simulink model "Radial_LV_Grid_CVR"  (R2022a)
settings: Solver=ode23t  StartTime=0.0  StopTime=10  MaxStep=0.1  RelTol=1e-3
libraries: spsLoadFlowBusLib x3, spsThreePhaseVIMeasurementLib x3, spsPower3phPhasorLib x2, spsThreePhasePISectionLineLib x1, spsThreePhaseDynamicLoadLib x1, spsThreePhaseProgrammableVoltageSourceLib x1, spsThreePhaseTransformerTwoWindingsLib x1, spspowerguiLib x1
settings Model: Creator=matm  LastModifiedBy=nikos
settings SolverCC: ShapePreserveControl=EnableAll  AlgebraicLoopSolver=TrustRegion  SolverResetMethod=Robust
settings DataIOCC: ReturnWorkspaceOutputs=off
settings DebuggingCC: SFMachineParentedDataDiag=warning  ArithmeticOperatorsInVariantConditions=warning
settings SFSimCC: SimUseLocalCustomCode=off  CustomCodeUndefinedFunction=UseInterfaceOnly
settings RTWCC: RTWUseLocalCustomCode=off
settings CodeAppCC: StateflowObjectComments=on
settings SimscapeCC: SimscapeNormalizeSystem=off

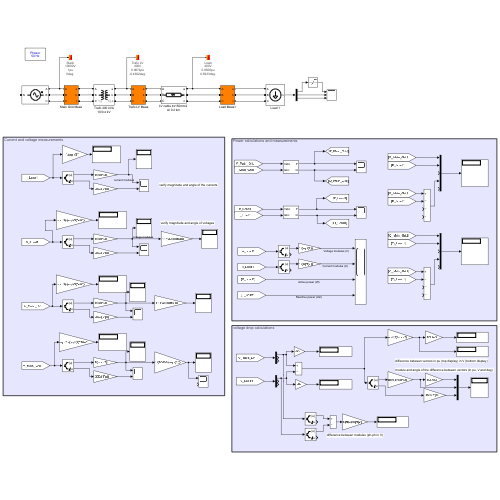
[thumbnail: Simulink's stored preview of the top-level diagram]
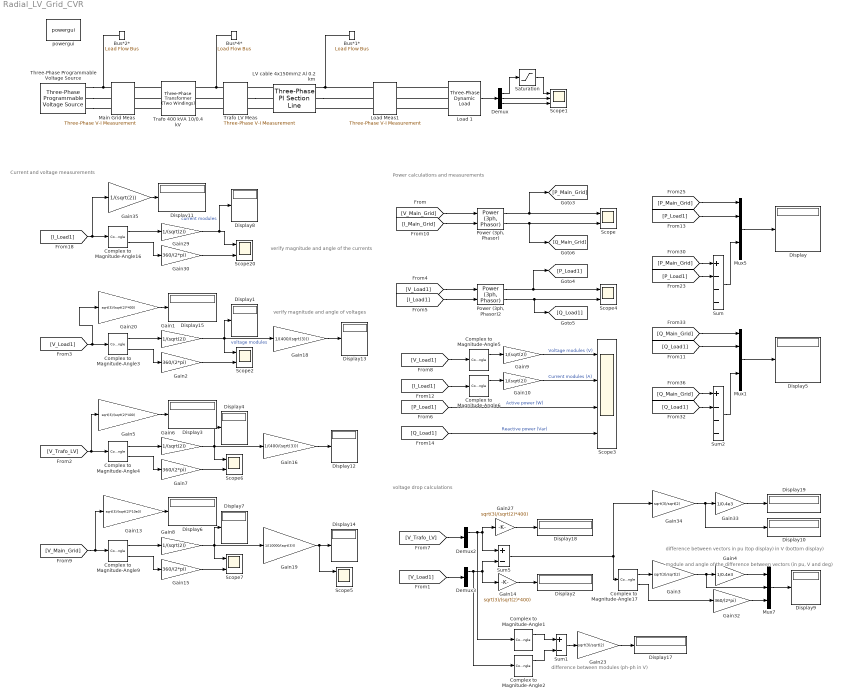
== system Radial_LV_Grid_CVR ==
  note: Power calculations and measurements
  note: voltage drop calculations
  note: difference between vectors in pu (top display) in V (bottom display)
  note: verify magnitude and angle of voltages
  note: verify magnitude and angle of the currents
  note: Current and voltage measurements
  note: difference between modules (ph-ph in V)
  note: module and angle of the difference between vectors (in pu, V and deg)
  Bus*1* : spsLoadFlowBusLib/Load Flow Bus  LConnTagsString=a  Phases=single  Connectors=on one side  ID=Load  Vbase=400  Vref=1  Vangle=0  VLF=0.9506  VLFb=1  VLFc=1  angleLF=0.5933  angleLFb=0  angleLFc=0
      settings: SourceProductBaseCode=PS
  Bus*2* : spsLoadFlowBusLib/Load Flow Bus  LConnTagsString=a  Phases=single  Connectors=on one side  ID=Slack  Vbase=10000  Vref=1  Vangle=0  VLF=1  VLFb=1  VLFc=1  angleLF=0  angleLFb=0  angleLFc=0
      settings: SourceProductBaseCode=PS
  Bus*4* : spsLoadFlowBusLib/Load Flow Bus  LConnTagsString=a  Phases=single  Connectors=on one side  ID=Trafo LV  Vbase=400  Vref=1  Vangle=0  VLF=0.9874  VLFb=1  VLFc=1  angleLF=-0.4362  angleLFb=0  angleLFc=0
      settings: SourceProductBaseCode=PS
  Complex to Magnitude-Angle{1..6,9,16..17} (9 alike) : ComplexToMagnitudeAngle
  Demux : Demux  Outputs=3
  Demux2 : Demux  Outputs=3
  Demux3 : Demux  Outputs=3
  Display{,1..15,17..19} (19 alike) : Display
  Gain{1,6,8..10,29,35} (7 alike) : Gain  Gain=1/(sqrt(2))
  Gain13 : Gain  Gain=sqrt(3)/(sqrt(2)*10e3)
  Gain{5,14,20,27} (4 alike) : Gain  Gain=sqrt(3)/(sqrt(2)*400)
  Gain{2,7,15,30,32} (5 alike) : Gain  Gain=360/(2*pi)
  Gain16 : Gain  Gain=1/(400/(sqrt(3)))
  Gain18 : Gain  Gain=1/(400/(sqrt(3)))
  Gain19 : Gain  Gain=1/(10000/(sqrt(3)))
  Gain23 : Gain  Gain=sqrt(3)/sqrt(2)
  Gain3 : Gain  Gain=sqrt(3)/sqrt(2)
  Gain33 : Gain  Gain=1/0.4e3
  Gain34 : Gain  Gain=sqrt(3)/sqrt(2)
  Gain4 : Gain  Gain=1/0.4e3
  LV cable 4x150mm2 Al 0.2 km : spsThreePhasePISectionLineLib/Three-Phase PI Section Line  LConnTagsString=a|b|c  RConnTagsString=A|B|C  Length=0.2  Frequency=50  Resistances=[ 0.207 0.83]  Inductances=[ 72e-3/(2*pi*50) 289e-3/(2*pi*50)]  Capacitances=[910e-09 411e-09]
  Load 1 : spsThreePhaseDynamicLoadLib/Three-Phase Dynamic Load  NominalVoltage=[ 0.4e3 50 ]  ActiveReactivePowers=[100000 100000]  PositiveSequence=[0.950611 0.593329]  ExternalControl=off  NpNq=[2 2]  TimeConstants="[0  0  0  0]"  MinimumVoltage=0.7  Tfilter=1e-4  LoadFlowParameters=[4 100000 0 0 100000]
      settings: SourceProductBaseCode=PS
  Load Meas1 : spsThreePhaseVIMeasurementLib/Three-Phase V-I Measurement  VoltageMeasurement=phase-to-ground  SetLabelV=on  LabelV=V_Load1  Vpu=off  VpuLL=off  CurrentMeasurement=yes  SetLabelI=on  LabelI=I_Load1  Ipu=off  Pbase=100e6  Vbase=500e3  OutputType=Complex  PhasorSimulation=on  PSBequivalent=0
  Main Grid Meas : spsThreePhaseVIMeasurementLib/Three-Phase V-I Measurement  VoltageMeasurement=phase-to-ground  SetLabelV=on  LabelV=V_Main_Grid  Vpu=off  VpuLL=off  CurrentMeasurement=yes  SetLabelI=on  LabelI=I_Main_Grid  Ipu=off  Pbase=100e6  Vbase=500e3  OutputType=Complex  PhasorSimulation=on  PSBequivalent=0
  Mux1 : Mux  Inputs=5
  Mux5 : Mux  Inputs=5
  Mux7 : Mux  Inputs=3
  "Power (3ph, Phasor)" : spsPower3phPhasorLib/Power (3ph, Phasor)
      settings: SourceProductBaseCode=PS
  "Power (3ph, Phasor)2" : spsPower3phPhasorLib/Power (3ph, Phasor)
      settings: SourceProductBaseCode=PS
  Saturation : Saturate  UpperLimit=1.15  LowerLimit=0.85
  Scope{,2,4..7,20} (7 alike) : Scope  NumInputPorts=2
  Scope1 : Scope  NumInputPorts=3
  Scope3 : Scope  NumInputPorts=4
  Sum : Sum  Inputs=+---
  Sum1 : Sum  Inputs=+-
  Sum2 : Sum  Inputs=+---
  Sum5 : Sum  Inputs=+-
  Three-Phase Programmable Voltage Source : spsThreePhaseProgrammableVoltageSourceLib/Three-Phase Programmable Voltage Source  PositiveSequence=[(10000)*1 0 50]  VariationEntity=Amplitude  VariationType=Table of time-amplitude pairs  VariationTypeAlt=Step  VariationStep=0.5  VariationRate=10  VariationMagnitude=0.3  VariationFrequency=2  VariationTiming=[1 2]  VariationPhaseA=off  Amplitudes=[1 0.99 0.98 0.97 0.96 0.95]  TimeValues=[0 1 2 3 4 5]  HarmonicGeneration=off  HarmonicA=[3 0.2 -25 0]  HarmonicB=[2 0.15 35 2]  Timing="[0.05  3]"  BusType=swing  Pref=0  Qref=0  Qmin=-inf  Qmax=inf
  Trafo 400 kVA 10/0.4 kV : spsThreePhaseTransformerTwoWindingsLib/Three-Phase Transformer (Two Windings)  Winding1Connection=Yg  Winding2Connection=Yg  CoreType=Three single-phase transformers  SetSaturation=off  Hysteresis=off  DataFile='hysteresis'  SetInitialFlux=off  Measurements=None  UNITS=pu  NominalPower=[ 400e3 , 50 ]  Winding1=[10000 0.005 0.019]  Winding2=[400 0.005 0.019]  Rm=500  Lm=500  L0=0.5  Saturation=[0 0;0.0024 1.2;1 1.52]  InitialFluxes=[0.8 -0.8 0.7]  BreakLoop=off  DiscreteSolver=Trapezoidal iterative  DataType=off  TransfoNumber=1
  Trafo LV Meas : spsThreePhaseVIMeasurementLib/Three-Phase V-I Measurement  VoltageMeasurement=phase-to-ground  SetLabelV=on  LabelV=V_Trafo_LV  Vpu=off  VpuLL=off  CurrentMeasurement=yes  SetLabelI=on  LabelI=I_Trafo_LV  Ipu=off  Pbase=100e6  Vbase=500e3  OutputType=Complex  PhasorSimulation=on  PSBequivalent=0
  powergui : spspowerguiLib/powergui  Priority=1  SimulationMode=Phasor  SampleTime=50e-6  frequency=50  Iterations=50  frequencyindice=50  Pbase=1e6  ErrMax=0.0001  UnitsV=kV  UnitsW=kW  buscounter=7  FunctionMessages=off  echomessages=off  EnableUseOfTLC=off  CurrentSourceSwitches=off  DisableSnubberDevices=off  DisableRonSwitches=off  DisableVfSwitches=off  DisplayEquations=off  AutomaticDiscreteSolvers=off  SolverType=Tustin/Backward Euler (TBE)  Interpol=off  ExternalGateDelay=off  methode=off  Ts=10  x0status=blocks  SPID=off  SwTol=0  HookPort=off  NonlinearTolerance=1e-4  nMaxIteration=100  ContinueOnMaxIteration=off  RestoreLinks=warning  ResistiveCurrentMeasurement=off  Frange=[0:2:500]  Ylog=off  Xlog=on  ShowGrid=off  save=off  variable=ZData  structure=ScopeData  ZoomFFT=off  StartTime=0.0  cycles=1  DisplayStyle=1  fundamental=60  FreqAxis=off  MaxFrequency=1000  frequencyindicesteady=1  RmsSteady=2  display=off
  wires:
  Load 1/1 -> Demux/1
  Demux/3 -> Scope1/3
  Demux/2 -> Scope1/2
  Demux/1 -> Saturation/1
  Saturation/1 -> Scope1/1
  "Power (3ph, Phasor)2"/1 -> [P_Load1], Scope4/1
  Sum2/1 -> Mux1/4
  [P_Main_Grid] -> Sum/1
  [P_Load1] -> Mux5/2
  Mux5/1 -> Display/1
  Gain27/1 -> Display18/1
  [P_Main_Grid] -> Mux5/1
  Sum/1 -> Mux5/4
  [Q_Load1] -> Sum2/2
  [Q_Main_Grid] -> Sum2/1
  [Q_Main_Grid] -> Mux1/1
  [Q_Load1] -> Mux1/2
  Mux1/1 -> Display5/1
  Complex to Magnitude-Angle3/2 -> Gain2/1
  [V_Main_Grid] -> Gain13/1, Complex to Magnitude-Angle9/1
  Gain3/1 -> Mux7/2, Gain4/1
  Complex to Magnitude-Angle9/2 -> Gain15/1
  Gain18/1 -> Display13/1
  Gain20/1 -> Display15/1
  Gain32/1 -> Mux7/3
  [P_Load1] -> Sum/2
  Gain23/1 -> Display17/1
  [V_Trafo_LV] -> Complex to Magnitude-Angle4/1, Gain5/1
  Gain33/1 -> Display19/1
  Sum1/1 -> Gain23/1
  Gain6/1 -> Gain16/1, Scope6/1, Display4/1
  Gain4/1 -> Mux7/1
  Demux2/1 -> Sum5/1, Gain27/1, Complex to Magnitude-Angle1/1
  Gain8/1 -> Scope7/1, Gain19/1, Display7/1
  Gain15/1 -> Scope7/2
  Gain14/1 -> Display2/1
  "Power (3ph, Phasor)"/1 -> Scope/1, [P_Main_Grid]
  Gain5/1 -> Display3/1
  Complex to Magnitude-Angle3/1 -> Gain1/1
  Gain19/1 -> Scope5/1, Display14/1
  Gain13/1 -> Display6/1
  [V_Load1] -> Complex to Magnitude-Angle3/1, Gain20/1
  [I_Load1] -> "Power (3ph, Phasor)2"/2
  Gain29/1 -> Scope20/1, Display8/1  "current modules"
  [V_Load1] -> Demux3/1
  Gain2/1 -> Scope2/2
  [I_Main_Grid] -> "Power (3ph, Phasor)"/2
  Complex to Magnitude-Angle2/1 -> Sum1/2
  Complex to Magnitude-Angle16/1 -> Gain29/1
  Gain7/1 -> Scope6/2
  Gain1/1 -> Scope2/1, Gain18/1, Display1/1  "voltage modules"
  Gain30/1 -> Scope20/2
  Complex to Magnitude-Angle17/2 -> Gain32/1
  Complex to Magnitude-Angle4/2 -> Gain7/1
  Mux7/1 -> Display9/1
  [V_Main_Grid] -> "Power (3ph, Phasor)"/1
  Complex to Magnitude-Angle4/1 -> Gain6/1
  Demux3/1 -> Gain14/1, Sum5/2, Complex to Magnitude-Angle2/1
  Complex to Magnitude-Angle1/1 -> Sum1/1
  Complex to Magnitude-Angle16/2 -> Gain30/1
  Gain35/1 -> Display11/1
  Gain16/1 -> Display12/1
  Gain34/1 -> Gain33/1, Display10/1
  Complex to Magnitude-Angle9/1 -> Gain8/1
  [V_Trafo_LV] -> Demux2/1
  "Power (3ph, Phasor)2"/2 -> [Q_Load1], Scope4/2
  [V_Load1] -> "Power (3ph, Phasor)2"/1
  "Power (3ph, Phasor)"/2 -> Scope/2, [Q_Main_Grid]
  Complex to Magnitude-Angle17/1 -> Gain3/1
  Sum5/1 -> Complex to Magnitude-Angle17/1, Gain34/1
  [I_Load1] -> Gain35/1, Complex to Magnitude-Angle16/1
  [P_Load1] -> Scope3/3  "Active power (W)"
  Gain9/1 -> Scope3/1  "Voltage modules (V)"
  [V_Load1] -> Complex to Magnitude-Angle5/1
  [I_Load1] -> Complex to Magnitude-Angle6/1
  Complex to Magnitude-Angle5/1 -> Gain9/1
  Complex to Magnitude-Angle6/1 -> Gain10/1
  Gain10/1 -> Scope3/2  "Current modules (A)"
  [Q_Load1] -> Scope3/4  "Reactive power (Var)"
  connections:
  Main Grid Meas/LConn1 -- Three-Phase Programmable Voltage Source/RConn1 -- Bus*2*/LConn1
  Three-Phase Programmable Voltage Source/RConn2 -- Main Grid Meas/LConn2
  Three-Phase Programmable Voltage Source/RConn3 -- Main Grid Meas/LConn3
  Trafo 400 kVA 10/0.4 kV/LConn3 -- Main Grid Meas/RConn3
  Trafo 400 kVA 10/0.4 kV/LConn1 -- Main Grid Meas/RConn1
  Trafo 400 kVA 10/0.4 kV/LConn2 -- Main Grid Meas/RConn2
  Trafo 400 kVA 10/0.4 kV/RConn1 -- Trafo LV Meas/LConn1 -- Bus*4*/LConn1
  Trafo LV Meas/LConn2 -- Trafo 400 kVA 10/0.4 kV/RConn2
  Trafo LV Meas/LConn3 -- Trafo 400 kVA 10/0.4 kV/RConn3
  LV cable 4x150mm2 Al 0.2 km/LConn1 -- Trafo LV Meas/RConn1
  Trafo LV Meas/RConn2 -- LV cable 4x150mm2 Al 0.2 km/LConn2
  LV cable 4x150mm2 Al 0.2 km/LConn3 -- Trafo LV Meas/RConn3
  LV cable 4x150mm2 Al 0.2 km/RConn1 -- Bus*1*/LConn1 -- Load Meas1/LConn1
  LV cable 4x150mm2 Al 0.2 km/RConn2 -- Load Meas1/LConn2
  Load Meas1/LConn3 -- LV cable 4x150mm2 Al 0.2 km/RConn3
  Load 1/LConn3 -- Load Meas1/RConn3
  Load 1/LConn2 -- Load Meas1/RConn2
  Load 1/LConn1 -- Load Meas1/RConn1
